simulink model "close_loop_system_retour_etat_cor"  (Simulink 7.7)
settings: Solver=ode45  StartTime=0.0  StopTime=10.0  RelTol=1e-3
values from neighbouring files (symbols this model uses):
  Jt = 0.002    [BE7_trame.m]
  K = place(sys.a, sys.b(:,1), Pc)    [BE7_trame.m]
  K_stat = MK_stat(1,1)    [BE7_trame.m]
  Kci = 1    [BE7_trame.m]
  Kcp = 1    [BE7_trame.m]
  Kcv = 0.0314    [BE7_trame.m]
  Ke = 0.2    [BE7_trame.m]
  Kg = 0.2    [BE7_trame.m]
  Le = 0.002    [BE7_trame.m]
  N = 300    [BE7_trame.m]
  Re = 2    [BE7_trame.m]
  sys = linmod('open_loop_system')    [BE7_trame.m]
libraries: simulink x2
settings Model: Creator=Anthony  LastModifiedBy=Anthony

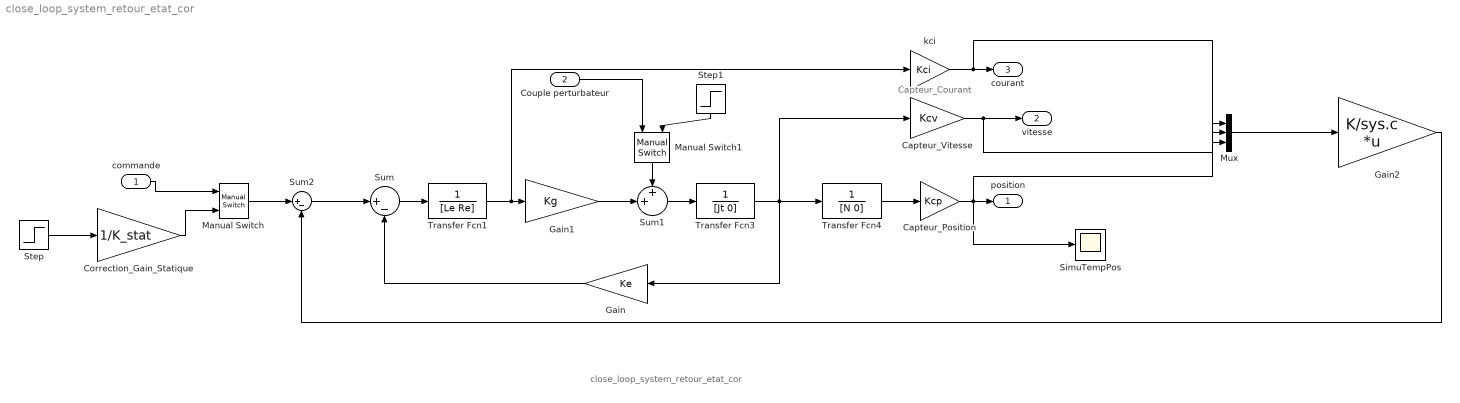
== system close_loop_system_retour_etat_cor ==
  note: close_loop_system_retour_etat_cor
  note: Capteur_Courant
  commande : Inport
  Couple perturbateur : Inport  Port=2
  Capteur_Position : Gain  Gain=Kcp  SaturateOnIntegerOverflow=on  OutDataTypeStr=Inherit: Same as input  ParamDataTypeStr=Inherit: Same as input
  Capteur_Vitesse : Gain  Gain=Kcv  SaturateOnIntegerOverflow=on  OutDataTypeStr=Inherit: Same as input  ParamDataTypeStr=Inherit: Same as input
  Correction_Gain_Statique : Gain  Gain=1/K_stat
  Gain : Gain  Gain=Ke  SaturateOnIntegerOverflow=on  OutDataTypeStr=Inherit: Same as input  ParamDataTypeStr=Inherit: Same as input
  Gain1 : Gain  Gain=Kg  SaturateOnIntegerOverflow=on  OutDataTypeStr=Inherit: Same as input  ParamDataTypeStr=Inherit: Same as input
  Gain2 : Gain  Gain=K/sys.c  Multiplication=Matrix(K*u)
  Manual Switch : simulink/Signal Routing/Manual Switch  SystemSampleTime=-1  sw=0  action=0  varsize=off
  Manual Switch1 : simulink/Signal Routing/Manual Switch  SystemSampleTime=-1  sw=0  action=0  varsize=off
  Mux : Mux  Inputs=3
  SimuTempPos : Scope
  Step : Step  Time=0  After=100  SampleTime=0
  Step1 : Step  Time=5  After=5  SampleTime=0
  Sum : Sum  Inputs=|+-  SaturateOnIntegerOverflow=on  InputSameDT=on  OutDataTypeStr=Inherit: Same as first input
  Sum1 : Sum  Inputs=++|  SaturateOnIntegerOverflow=on  InputSameDT=on  OutDataTypeStr=Inherit: Same as first input
  Sum2 : Sum  Inputs=|+-
  Transfer Fcn1 : TransferFcn  Denominator=[Le Re]
  Transfer Fcn3 : TransferFcn  Denominator=[Jt 0]
  Transfer Fcn4 : TransferFcn  Denominator=[N 0]
  kci : Gain  Gain=Kci  SaturateOnIntegerOverflow=on  OutDataTypeStr=Inherit: Same as input  ParamDataTypeStr=Inherit: Same as input
  position : Outport
  vitesse : Outport  Port=2
  courant : Outport  Port=3
  wires:
  Sum/1 -> Transfer Fcn1/1
  Transfer Fcn1/1 -> Gain1/1, kci/1
  Transfer Fcn3/1 -> Capteur_Vitesse/1, Transfer Fcn4/1, Gain/1
  Gain/1 -> Sum/2
  Transfer Fcn4/1 -> Capteur_Position/1
  Gain1/1 -> Sum1/2
  Sum1/1 -> Transfer Fcn3/1
  commande/1 -> Manual Switch/1
  Gain2/1 -> Sum2/2
  Step/1 -> Correction_Gain_Statique/1
  Manual Switch/1 -> Sum2/1
  Sum2/1 -> Sum/1
  Step1/1 -> Manual Switch1/2
  Couple perturbateur/1 -> Manual Switch1/1
  Manual Switch1/1 -> Sum1/1
  Capteur_Position/1 -> SimuTempPos/1, Mux/1, position/1
  kci/1 -> courant/1, Mux/3
  Mux/1 -> Gain2/1
  Capteur_Vitesse/1 -> vitesse/1, Mux/2
  Correction_Gain_Statique/1 -> Manual Switch/2
